simulink model "Stan_Ilya_314_4_1"  (R2018a)
settings: Solver=VariableStepAuto  StartTime=0.0  StopTime=7  RelTol=1e-3
settings Model: Creator=ilya  LastModifiedBy=ilya

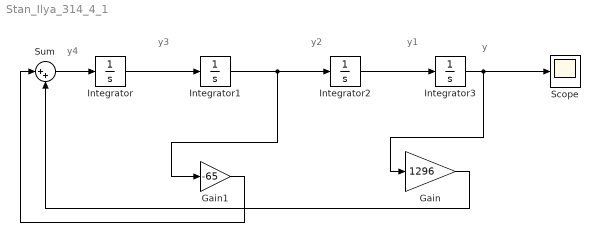
== system Stan_Ilya_314_4_1 ==
  note: y
  note: y1
  note: y2
  note: y3
  note: y4
  Gain : Gain  Gain=1296
  Gain1 : Gain  Gain=-65
  Integrator : Integrator  InitialCondition=-985
  Integrator1 : Integrator  InitialCondition=64
  Integrator2 : Integrator  InitialCondition=-7
  Integrator3 : Integrator  InitialCondition=4
  Scope : Scope
  Sum : Sum  Inputs=|++
  wires:
  Integrator/1 -> Integrator1/1
  Integrator1/1 -> Gain1/1, Integrator2/1
  Integrator2/1 -> Integrator3/1
  Integrator3/1 -> Scope/1, Gain/1
  Sum/1 -> Integrator/1
  Gain/1 -> Sum/2
  Gain1/1 -> Sum/1
